simulink model "intensity"  (R2020b)
settings: Solver=FixedStepAuto  StartTime=0.0  StopTime=stop_time  FixedStep=1  RelTol=1e-3
InitFcn:
  | test_FFT_to_gain_init
StopFcn:
  | test_FFT_to_gain_stop
values from neighbouring files (symbols this model uses):
  num_bins = FFTsize/2 + 1    (= 129)    [intensity_sim_init.m]
libraries: simulink x5
settings Model: Creator=t96f346  LastModifiedBy=t96f346
settings DataIOCC: SaveOutput=off  SaveTime=off

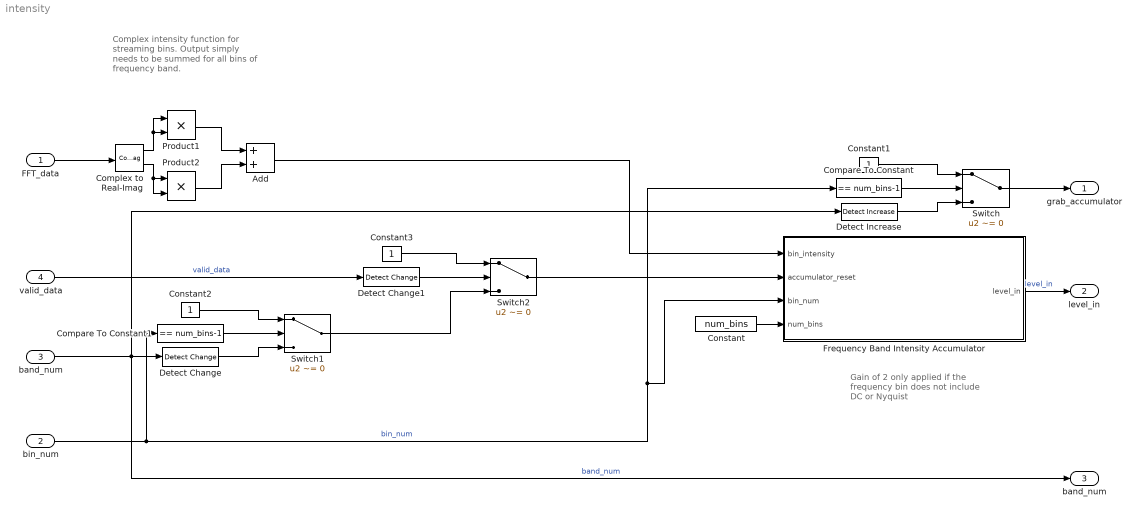
== system intensity ==
  note: Gain of 2 only applied if the frequency bin does not include DC or Nyquist
  note: Complex intensity function for streaming bins. Output simply needs to be summed for all bins of frequency band.
  FFT_data : Inport  OutDataTypeStr=fixdt(1,40,32)  PortDimensions=[1 1]  SampleTime=[1,0]
      settings: SignalType=complex
  bin_num : Inport  Port=2  OutDataTypeStr=uint8  PortDimensions=1  SampleTime=[1,0]
  band_num : Inport  Port=3  OutDataTypeStr=uint8  PortDimensions=1  SampleTime=[1,0]
  "valid_data " : Inport  Port=4  OutDataTypeStr=boolean  PortDimensions=[1 1]  SampleTime=[1,0]
  Add : Sum  OutDataTypeStr=fixdt(1,Wbits,Fbits)
  Compare To Constant : simulink/Logic and Bit Operations/Compare To Constant  relop===  const=num_bins-1  OutDataTypeStr=boolean
  Compare To Constant1 : simulink/Logic and Bit Operations/Compare To Constant  relop===  const=num_bins-1  OutDataTypeStr=boolean
  Complex to Real-Imag : ComplexToRealImag
  Constant : Constant  Value=num_bins  OutDataTypeStr=uint8  SampleTime=-1
  Constant1 : Constant  OutDataTypeStr=boolean  SampleTime=-1
  Constant2 : Constant  OutDataTypeStr=boolean  SampleTime=-1
  Constant3 : Constant  OutDataTypeStr=boolean  SampleTime=-1
  Detect Change : simulink/Logic and Bit Operations/Detect Change  vinit=1  OutDataTypeStr=boolean
  Detect Change1 : simulink/Logic and Bit Operations/Detect Change  vinit=1  OutDataTypeStr=boolean
  Detect Increase : simulink/Logic and Bit Operations/Detect Increase  vinit=1  OutDataTypeStr=boolean
  Frequency Band Intensity Accumulator : MATLAB Function  TreatAsAtomicUnit=on
  Product1 : Product  OutDataTypeStr=fixdt(1,Wbits,Fbits)
  Product2 : Product  OutDataTypeStr=fixdt(1,Wbits,Fbits)
  Switch : Switch  Criteria=u2 ~= 0
  Switch1 : Switch  Criteria=u2 ~= 0
  Switch2 : Switch  Criteria=u2 ~= 0
  grab_accumulator : Outport  OutDataTypeStr=boolean  PortDimensions=1  SampleTime=[1,0]  VectorParamsAs1DForOutWhenUnconnected=off
  level_in : Outport  Port=2  OutDataTypeStr=fixdt(1,40,32)  PortDimensions=1  SampleTime=[1,0]
  "band_num " : Outport  Port=3  OutDataTypeStr=uint8  PortDimensions=1  SampleTime=[1,0]
  wires:
  Switch2/1 -> Frequency Band Intensity Accumulator/2(accumulator_reset)
  Detect Change1/1 -> Switch2/2
  Constant3/1 -> Switch2/1
  "valid_data "/1 -> Detect Change1/1  "valid_data"
  Switch1/1 -> Switch2/3
  Detect Change/1 -> Switch1/3
  Compare To Constant1/1 -> Switch1/2
  Constant2/1 -> Switch1/1
  band_num/1 -> "band_num "/1, Detect Increase/1, Detect Change/1  "band_num"
  Switch/1 -> grab_accumulator/1
  Constant1/1 -> Switch/1
  bin_num/1 -> Compare To Constant1/1, Frequency Band Intensity Accumulator/3(bin_num), Compare To Constant/1  "bin_num"
  Compare To Constant/1 -> Switch/2
  Constant/1 -> Frequency Band Intensity Accumulator/4(num_bins)
  Detect Increase/1 -> Switch/3
  Frequency Band Intensity Accumulator/1(level_in) -> level_in/1  "level_in"
  FFT_data/1 -> Complex to Real-Imag/1
  Add/1 -> Frequency Band Intensity Accumulator/1(bin_intensity)
  Product1/1 -> Add/1
  Complex to Real-Imag/2 -> Product2/2, Product2/1
  Complex to Real-Imag/1 -> Product1/1, Product1/2
  Product2/1 -> Add/2

== matlab function intensity/Frequency Band Intensity Accumulator ==
  data: bin_intensity input; level_in output fixdt(1,Wbits,Fbits); accumulator_reset input; bin_num input; num_bins input
function level_in = accumulate_band(bin_intensity, accumulator_reset, bin_num, num_bins)

% Accumulates the bin intensities until a new frequency band is detected.
% Takes in the current frequency bin intensity, an accumulator reset
% control signal, bin number and number of frequency bins. If the 
% accumulator_reset is true, the sum is reset starting with the current 
% frequency bin intensity. Unless a DC or Nyquist bin is detected, a
% logical shift left is executed to apply a gain of two to the current
% bin_intensity, which accounts for negative frequencies.

persistent total;

if isempty(total)
    total = fi(0,1,40,32);
end

if bin_num == 0 || bin_num == num_bins-1
    dc_nyquist = true;
else
    dc_nyquist = false;
end

if accumulator_reset == true && dc_nyquist == true
    total = fi(bin_intensity,1,40,32);
    level_in = total;
elseif accumulator_reset == true && dc_nyquist == false
    total = bitsll(fi(bin_intensity,1,40,32),fi(1));
    level_in = total;
elseif accumulator_reset == false && dc_nyquist == true
    total = fi(total + fi(bin_intensity,1,40,32),1,40,32);
    level_in = total;
elseif accumulator_reset == false && dc_nyquist == false
    total = fi(total + bitsll(fi(bin_intensity,1,40,32),fi(1)),1,40,32);
    level_in = total;
else
    total = fi(0,1,40,32);
    error('Incorrect Logic in accumulate_band function!');
end
